simulink model "boost_and_two_level_bridge_rtlab_2_sc_console"  (Simulink 8.4)
settings: Solver=ode3  SolverMode=SingleTasking  StartTime=0.0  StopTime=inf  FixedStep=2e-05  RelTol=1e-3
PostLoadFcn:
  | Ts = 20e-6;
InitFcn:
  | Ts = 20e-6;
libraries: opal_lib x6, simulink x2, efs_cpuhilios_crtl_lib x1
settings Model: ARTEMISmethode_block_infos=$$__separator__$$boost_and_two_level_bridge_rtlab/ARTEMIS Guide$$__separator__$$  Creator=PYRobert  LastModifiedBy=jiang  BufferReuse=off
settings DataIOCC: SaveOutput=off  SignalLogging=off  SaveTime=off  SignalLoggingName=sigsOut
settings OptimizationCC: BlockReduction=off  OptimizeBlockIOStorage=off  BufferReuse=off  GlobalBufferReuse=off  ExpressionFolding=off  LocalBlockOutputs=off  InitFltsAndDblsToZero=on
settings DebuggingCC: SaveWithParameterizedLinksMsg=none  SignalResolutionControl=TryResolveAllWithWarning  SolverPrmCheckMsg=none  MultiTaskDSMMsg=warning  MultiTaskCondExecSysMsg=none
settings HardwareCC: TargetEndianess=LittleEndian  TargetHWDeviceType=MATLAB Host  ProdEqTarget=off
settings RTWCC: GenCodeOnly=on  IncludeERTFirstTime=on
settings GRTTargetCC: TargetFcnLib=ansi_tfl_tmw.mat
settings ConfigurationSet: Description=SimMechanics 2G

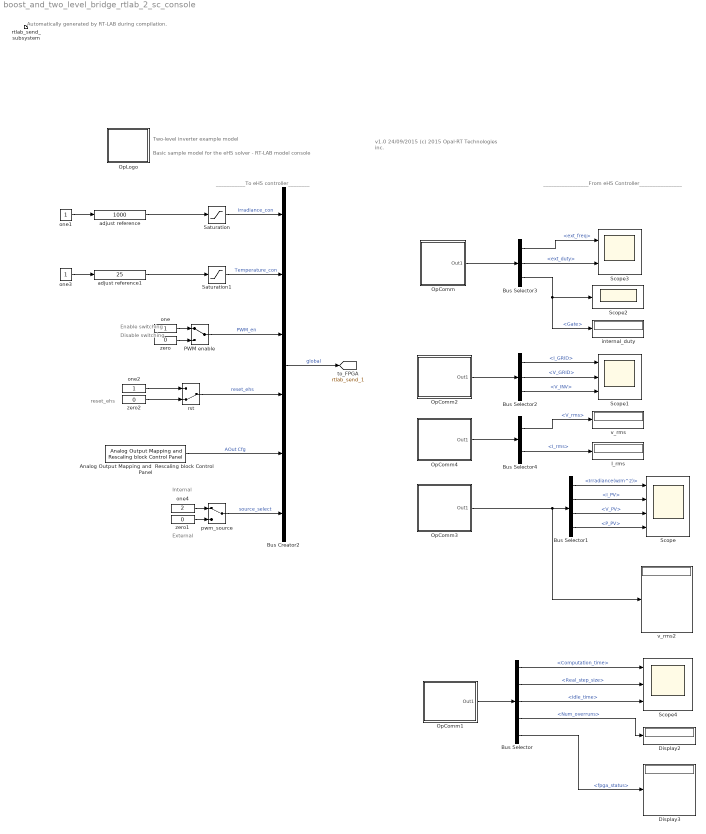
== system boost_and_two_level_bridge_rtlab_2_sc_console ==
  note: reset_ehs
  note: Basic sample model for the eHS solver - RT-LAB model console
  note: Two-level inverter example model
  note: v1.0 24/09/2015
      | (c) 2015 Opal-RT Technologies inc.
  note: Disable switching
  note: Enable switching
  note: _________________From eHS Controller________________
  note: ___________To eHS controller________
  note: Internal
  note: External
  note: Automatically generated by RT-LAB during compilation.
  Analog Output Mapping and  Rescaling block Control Panel : efs_cpuhilios_crtl_lib/Analog Output Mapping and  Rescaling block Control Panel  NbChannels=32  SigNames={'eHS.Y01' 'eHS.Y02' 'eHS.Y03' 'eHS.Y04' 'eHS.Y05' 'eHS.Y06' 'eHS.Y07' 'eHS.Y08' 'eHS.Y09' 'eHS.Y10' 'eHS.Y11' 'eHS.Y12' 'eHS.Y13' 'eHS.Y14' 'eHS.Y15' 'eHS.Y16' 'eHS.Y17' 'eHS.Y18' 'eHS.Y19' 'eHS.Y20' 'eHS.Y21' 'eHS.Y22' 'eHS.Y23' 'eHS.Y24' 'eHS.Y25' 'eHS.Y26' 'eHS.Y27' 'eHS.Y28' 'eHS.Y29' 'eHS.Y30' 'eHS.Y31' 'eHS.Y32'}  NbUsrAOut=16  signalch0=User2  signalch1=User1  signalch2=User5  signalch3=User6  signalch4=User6  signalch5=eHS.Y10  signalch6=eHS.Y02  signalch7=eHS.Y04  signalch8=eHS.Y13  signalch9=eHS.Y14  signalch10=eHS.Y01  signalch11=eHS.Y03  signalch12=User1  signalch13=User2  signalch14=User3  signalch15=User4  signalch16=User1  signalch17=User2  signalch18=User3  signalch19=User4  signalch20=User5  signalch21=User6  signalch22=User7  signalch23=User7  signalch24=User9  signalch25=User10  signalch26=User11  signalch27=User12  signalch28=User13  signalch29=User14  signalch30=User15  signalch31=User16  gain0=0.0066  gain1=0.33  gain2=0.066  gain3=0.0041250  gain4=0.0048529  gain5=1  gain6=0.005  gain7=0.005  gain8=0.1  gain9=0.1  gain10=0.1  gain11=0.1  gain12=.005  gain13=.1  gain14=.1  gain15=.1  gain16=1  gain17=1  gain18=1  gain19=1  gain20=1  gain21=1  gain22=1  gain23=1  gain24=1  gain25=1  gain26=1  gain27=1  gain28=1  gain29=1  gain30=1  gain31=1  offset0=0  offset1=0  offset2=1.65  offset3=1.6500  offset4=1.6500  offset5=0  offset6=0  offset7=0  offset8=0  offset9=0  offset10=0  offset11=0  offset12=0  offset13=0  offset14=0  offset15=0  offset16=0  offset17=0  offset18=0  offset19=0  offset20=0  offset21=0  offset22=0  offset23=0  offset24=0  offset25=0  offset26=0  offset27=0  offset28=0  offset29=0  offset30=0  offset31=0  max0=3.3  max1=3.3  max2=3.3  max3=3.3  max4=3.3  max5=5  max6=5  max7=5  max8=5  max9=5  max10=5  max11=5  max12=16  max13=16  max14=16  max15=16  max16=16  max17=16  max18=16  max19=16  max20=16  max21=16  max22=16  max23=16  max24=16  max25=16  max26=16  max27=16  max28=16  max29=16  max30=16  max31=16  min0=0  min1=0  min2=0  min3=0  min4=0  min5=-5  min6=-5  min7=-5  min8=-5  min9=-5  min10=-5  min11=-5  min12=-16  min13=-16  min14=-16  min15=-16  min16=-16  min17=-16  min18=-16  min19=-16  min20=-16  min21=-16  min22=-16  min23=-16  min24=-16  min25=-16  min26=-16  min27=-16  min28=-16  min29=-16  min30=-16  min31=-16  map=[ 49 48 52 53 53 9 1 3 12 13 0 2 48 49 50 51 48 49 50 51 52 53 54 54 56 57 58 59 60 61 62 63 ]
      link override Display2: Decimation=12500
  Bus Creator2 : BusCreator  Inputs=6
  Bus Selector : BusSelector  OutputSignals=Computation_time,Real_step_size,Idle_time,Num_overruns,fpga_status
  Bus Selector1 : BusSelector  OutputSignals=Irradiance(w/m^2),I_PV,V_PV,P_PV
  Bus Selector2 : BusSelector  OutputSignals=I_GRID,V_GRID,V_INV
  Bus Selector3 : BusSelector  OutputSignals=digital_in.ext_freq,digital_in.ext_duty,Gate
  Bus Selector4 : BusSelector  OutputSignals=V_rms,I_rms
  Display2 : Display
      settings: Decimation=12500
  Display3 : Display
      settings: Decimation=12500
  I_rms : Display
      settings: Decimation=12500
  OpComm : Subsystem
      mask init:
      | opmaskdisplay('maskdisplay_block',gcb,'disp(''OpComm'')');
      mask Display:
      | patch([0 0.5 0.7 0],[1 1 0 0],[0.7 0.75 0.9]);
      | patch([1 0.53 0.73 1],[1 1 0 0],[1 0.8 0.7]);
      | plot([0 0 1 1 0],[0 1 1 0 0]);
      | disp('OpComm')
  OpComm1 : Subsystem
      mask init:
      | opmaskdisplay('maskdisplay_block',gcb,'disp(''OpComm'')');
      mask Display:
      | patch([0 0.5 0.7 0],[1 1 0 0],[0.7 0.75 0.9]);
      | patch([1 0.53 0.73 1],[1 1 0 0],[1 0.8 0.7]);
      | plot([0 0 1 1 0],[0 1 1 0 0]);
      | disp('OpComm')
  OpComm2 : Subsystem
      mask init:
      | opmaskdisplay('maskdisplay_block',gcb,'disp(''OpComm'')');
      mask Display:
      | patch([0 0.5 0.7 0],[1 1 0 0],[0.7 0.75 0.9]);
      | patch([1 0.53 0.73 1],[1 1 0 0],[1 0.8 0.7]);
      | plot([0 0 1 1 0],[0 1 1 0 0]);
      | disp('OpComm')
  OpComm3 : Subsystem
      mask init:
      | opmaskdisplay('maskdisplay_block',gcb,'disp(''OpComm'')');
      mask Display:
      | patch([0 0.5 0.7 0],[1 1 0 0],[0.7 0.75 0.9]);
      | patch([1 0.53 0.73 1],[1 1 0 0],[1 0.8 0.7]);
      | plot([0 0 1 1 0],[0 1 1 0 0]);
      | disp('OpComm')
  OpComm4 : Subsystem
      mask init:
      | opmaskdisplay('maskdisplay_block',gcb,'disp(''OpComm'')');
      mask Display:
      | patch([0 0.5 0.7 0],[1 1 0 0],[0.7 0.75 0.9]);
      | patch([1 0.53 0.73 1],[1 1 0 0],[1 0.8 0.7]);
      | plot([0 0 1 1 0],[0 1 1 0 0]);
      | disp('OpComm')
  OpLogo : Subsystem
      mask Display:
      | opLogo = imread('efsOpLogo.tif','tif');
      | image(opLogo(:,:,1:3));
  PWM enable : ManualSwitch
  Saturation : Saturate  UpperLimit=1000  LowerLimit=0
  Saturation1 : Saturate  UpperLimit=60  LowerLimit=-10
  Scope : Scope  NumInputPorts=4
      settings: YMin=-5~-5~-5~-5  YMax=5~5~5~5  Decimation=100  SampleInput=on  SampleTime=2e-3
  Scope1 : Scope  NumInputPorts=3
      settings: YMin=-500~-400~-800  YMax=500~400~800  SaveName=ScopeData2  SampleInput=on  SampleTime=1e-3
  Scope2 : Scope
      settings: YMin=0  YMax=1  SaveName=ScopeData3  MaxDataPoints=10000  SampleInput=on  SampleTime=2e-4
  Scope3 : Scope  NumInputPorts=2
      settings: YMin=-5~-5  YMax=5~5  SaveName=ScopeData4  MaxDataPoints=100000  SampleInput=on  SampleTime=1e-3
  Scope4 : Scope  NumInputPorts=3
      settings: YMin=-5~-5~-5  YMax=5~5~5  SaveName=ScopeData5  SampleInput=on  SampleTime=5e-2
  adjust reference : simulink/Math Operations/Slider Gain  low=0  gain=1000  high=1000
  adjust reference1 : simulink/Math Operations/Slider Gain  low=0  gain=25  high=60
  internal_duty : Display
      settings: Decimation=12500
  one{,1..3} (4 alike) : Constant
  one4 : Constant  Value=2
  pwm_source : ManualSwitch
  rst : ManualSwitch  CurrentSetting=0
  rtlab_send_subsystem : Subsystem  Priority=-100
      mask Display: text(0,0,'');
  v_rms : Display
      settings: Decimation=12500
  v_rms2 : Display
      settings: Decimation=12500
  zero : Constant  Value=0
  zero1 : Constant  Value=0
  zero2 : Constant  Value=0
  tag scope: rtlab_send_1=global
  wires:
  Bus Selector4/2 -> I_rms/1  "<I_rms>"
  Bus Selector4/1 -> v_rms/1  "<V_rms>"
  OpComm4/1(Out1) -> Bus Selector4/1
  Bus Selector/5 -> Display3/1  "<fpga_status>"
  Bus Selector3/3 -> Scope2/1, internal_duty/1  "<Gate>"
  Bus Selector3/2 -> Scope3/2  "<ext_duty>"
  Bus Selector3/1 -> Scope3/1  "<ext_freq>"
  OpComm/1(Out1) -> Bus Selector3/1
  Bus Selector2/3 -> Scope1/3  "<V_INV>"
  Bus Selector2/1 -> Scope1/1  "<I_GRID>"
  Bus Selector2/2 -> Scope1/2  "<V_GRID>"
  OpComm2/1(Out1) -> Bus Selector2/1
  Bus Selector1/3 -> Scope/3  "<V_PV>"
  Bus Selector1/4 -> Scope/4  "<P_PV>"
  Bus Selector1/2 -> Scope/2  "<I_PV>"
  Bus Selector1/1 -> Scope/1  "<Irradiance(w/m^2)>"
  OpComm3/1(Out1) -> v_rms2/1, Bus Selector1/1
  OpComm1/1(Out1) -> Bus Selector/1
  pwm_source/1 -> Bus Creator2/6  "source_select"
  one4/1 -> pwm_source/1
  zero1/1 -> pwm_source/2
  Analog Output Mapping and  Rescaling block Control Panel/1 -> Bus Creator2/5  "AOut Cfg"
  Bus Selector/1 -> Scope4/1  "<Computation_time>"
  Bus Selector/4 -> Display2/1  "<Num_overruns>"
  Bus Selector/2 -> Scope4/2  "<Real_step_size>"
  Bus Selector/3 -> Scope4/3  "<Idle_time>"
  Saturation1/1 -> Bus Creator2/2  "Temperature_con"
  Saturation/1 -> Bus Creator2/1  "Irradiance_con"
  adjust reference1/1 -> Saturation1/1
  adjust reference/1 -> Saturation/1
  one3/1 -> adjust reference1/1
  one1/1 -> adjust reference/1
  one2/1 -> rst/1
  zero2/1 -> rst/2
  rst/1 -> Bus Creator2/4  "reset_ehs"
  one/1 -> PWM enable/1
  zero/1 -> PWM enable/2
  PWM enable/1 -> Bus Creator2/3  "PWM_en"
  Bus Creator2/1 -> [rtlab_send_1]  "global"

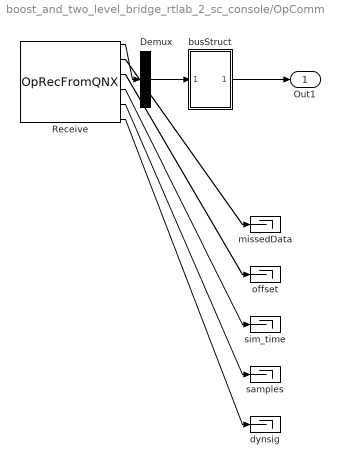
== system boost_and_two_level_bridge_rtlab_2_sc_console/OpComm ==
  Demux : Demux  Outputs=[4]
  Receive : opal_lib/Communication/OpRecFromQNX  Node_num=1  Acqu_Group=1  Data_Width=4  Synchronization=on  Interpolation=on  Threshold=1.0  modelname=boost_and_two_level_bridge_rtlab.mdl  sampletime=2e-05
  busStruct : Subsystem
  dynsig : Terminator
  missedData : Terminator
  offset : Terminator
  samples : Terminator
  sim_time : Terminator
  Out1 : Outport
  wires:
  Demux/1 -> busStruct/1(In1)
  busStruct/1(Out1) -> Out1/1
  Receive/1 -> Demux/1
  Receive/6 -> dynsig/1
  Receive/5 -> samples/1
  Receive/4 -> sim_time/1
  Receive/3 -> offset/1
  Receive/2 -> missedData/1

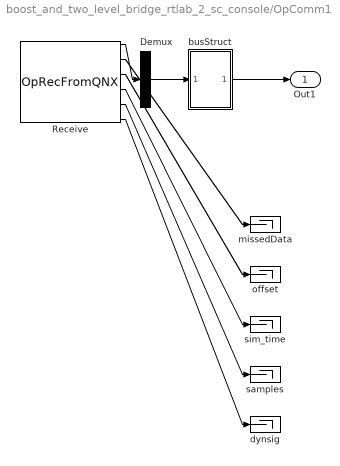
== system boost_and_two_level_bridge_rtlab_2_sc_console/OpComm1 ==
  Demux : Demux  Outputs=[8]
  Receive : opal_lib/Communication/OpRecFromQNX  Node_num=1  Acqu_Group=2  Data_Width=8  Synchronization=on  Interpolation=on  Threshold=1.0  modelname=boost_and_two_level_bridge_rtlab.mdl  sampletime=2e-05
  busStruct : Subsystem
  dynsig : Terminator
  missedData : Terminator
  offset : Terminator
  samples : Terminator
  sim_time : Terminator
  Out1 : Outport
  wires:
  Demux/1 -> busStruct/1(In1)
  busStruct/1(Out1) -> Out1/1
  Receive/1 -> Demux/1
  Receive/6 -> dynsig/1
  Receive/5 -> samples/1
  Receive/4 -> sim_time/1
  Receive/3 -> offset/1
  Receive/2 -> missedData/1

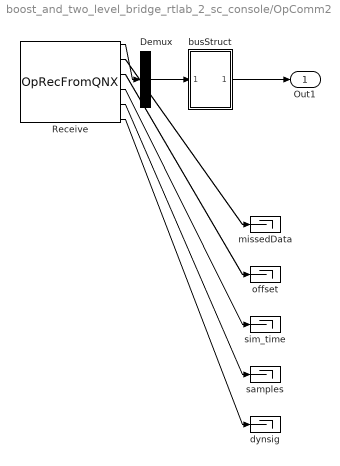
== system boost_and_two_level_bridge_rtlab_2_sc_console/OpComm2 ==
  Demux : Demux  Outputs=[3]
  Receive : opal_lib/Communication/OpRecFromQNX  Node_num=1  Acqu_Group=4  Data_Width=3  Synchronization=on  Interpolation=on  Threshold=1.0  modelname=boost_and_two_level_bridge_rtlab.mdl  sampletime=2e-05
  busStruct : Subsystem
  dynsig : Terminator
  missedData : Terminator
  offset : Terminator
  samples : Terminator
  sim_time : Terminator
  Out1 : Outport
  wires:
  Demux/1 -> busStruct/1(In1)
  busStruct/1(Out1) -> Out1/1
  Receive/1 -> Demux/1
  Receive/6 -> dynsig/1
  Receive/5 -> samples/1
  Receive/4 -> sim_time/1
  Receive/3 -> offset/1
  Receive/2 -> missedData/1

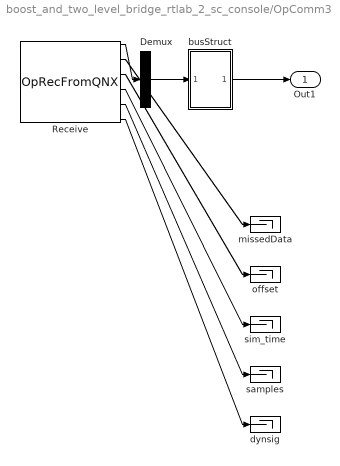
== system boost_and_two_level_bridge_rtlab_2_sc_console/OpComm3 ==
  Demux : Demux  Outputs=[6]
  Receive : opal_lib/Communication/OpRecFromQNX  Node_num=1  Acqu_Group=3  Data_Width=6  Synchronization=on  Interpolation=on  Threshold=1.0  modelname=boost_and_two_level_bridge_rtlab.mdl  sampletime=2e-05
  busStruct : Subsystem
  dynsig : Terminator
  missedData : Terminator
  offset : Terminator
  samples : Terminator
  sim_time : Terminator
  Out1 : Outport
  wires:
  Demux/1 -> busStruct/1(In1)
  busStruct/1(Out1) -> Out1/1
  Receive/1 -> Demux/1
  Receive/6 -> dynsig/1
  Receive/5 -> samples/1
  Receive/4 -> sim_time/1
  Receive/3 -> offset/1
  Receive/2 -> missedData/1

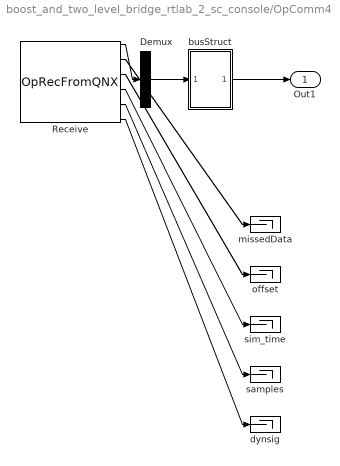
== system boost_and_two_level_bridge_rtlab_2_sc_console/OpComm4 ==
  Demux : Demux  Outputs=[2]
  Receive : opal_lib/Communication/OpRecFromQNX  Node_num=1  Acqu_Group=5  Data_Width=2  Synchronization=on  Interpolation=on  Threshold=1.0  modelname=boost_and_two_level_bridge_rtlab.mdl  sampletime=2e-05
  busStruct : Subsystem
  dynsig : Terminator
  missedData : Terminator
  offset : Terminator
  samples : Terminator
  sim_time : Terminator
  Out1 : Outport
  wires:
  Demux/1 -> busStruct/1(In1)
  busStruct/1(Out1) -> Out1/1
  Receive/1 -> Demux/1
  Receive/6 -> dynsig/1
  Receive/5 -> samples/1
  Receive/4 -> sim_time/1
  Receive/3 -> offset/1
  Receive/2 -> missedData/1

== system boost_and_two_level_bridge_rtlab_2_sc_console/OpLogo ==

== system boost_and_two_level_bridge_rtlab_2_sc_console/rtlab_send_subsystem ==
  Subsystem6 : Subsystem
  wires:
  [rtlab_send_1] -> Subsystem6/1(In1)

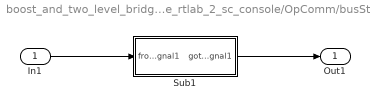
== system boost_and_two_level_bridge_rtlab_2_sc_console/OpComm/busStruct ==
  In1 : Inport
  Sub1 : Subsystem
  Out1 : Outport
  wires:
  Sub1/1(goto_signal1) -> Out1/1
  In1/1 -> Sub1/1(from_signal1)

== system boost_and_two_level_bridge_rtlab_2_sc_console/OpComm1/busStruct ==
  In1 : Inport
  Sub1 : Subsystem
  Out1 : Outport
  wires:
  Sub1/1(goto_signal1) -> Out1/1
  In1/1 -> Sub1/1(from_signal1)

== system boost_and_two_level_bridge_rtlab_2_sc_console/OpComm2/busStruct ==
  In1 : Inport
  Sub1 : Subsystem
  Out1 : Outport
  wires:
  Sub1/1(goto_signal1) -> Out1/1
  In1/1 -> Sub1/1(from_signal1)

== system boost_and_two_level_bridge_rtlab_2_sc_console/OpComm3/busStruct ==
  In1 : Inport
  Sub1 : Subsystem
  Out1 : Outport
  wires:
  Sub1/1(goto_signal1) -> Out1/1
  In1/1 -> Sub1/1(from_signal1)

== system boost_and_two_level_bridge_rtlab_2_sc_console/OpComm4/busStruct ==
  In1 : Inport
  Sub1 : Subsystem
  Out1 : Outport
  wires:
  Sub1/1(goto_signal1) -> Out1/1
  In1/1 -> Sub1/1(from_signal1)

== system boost_and_two_level_bridge_rtlab_2_sc_console/rtlab_send_subsystem/Subsystem6 ==
  In1 : Inport  PortDimensions=165
  Mux : Mux  Inputs=1
  Send6 : opal_lib/Communication/OpSendPar ToQNX  Node_num=1  modelname=boost_and_two_level_bridge_rtlab
  wires:
  Mux/1 -> Send6/1
  In1/1 -> Mux/1

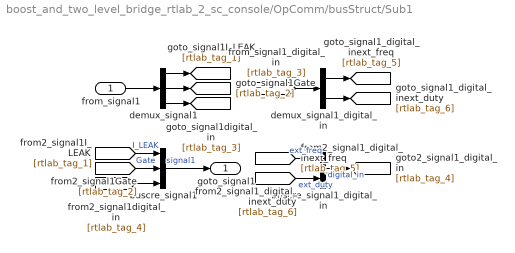
== system boost_and_two_level_bridge_rtlab_2_sc_console/OpComm/busStruct/Sub1 ==
  from_signal1 : Inport
  buscre_signal1 : BusCreator  Inputs=3
  buscre_signal1_digital_in : BusCreator  Inputs=2
  demux_signal1 : Demux  Outputs="[1  1  2]"
  demux_signal1_digital_in : Demux  Outputs="[1  1]"
  goto_signal1 : Outport
  wires:
  buscre_signal1_digital_in/1 -> [rtlab_tag_4]  "digital_in"
  [rtlab_tag_6] -> buscre_signal1_digital_in/2  "ext_duty"
  [rtlab_tag_5] -> buscre_signal1_digital_in/1  "ext_freq"
  demux_signal1_digital_in/2 -> [rtlab_tag_6]
  demux_signal1_digital_in/1 -> [rtlab_tag_5]
  [rtlab_tag_3] -> demux_signal1_digital_in/1
  buscre_signal1/1 -> goto_signal1/1  "signal1"
  [rtlab_tag_4] -> buscre_signal1/3
  [rtlab_tag_2] -> buscre_signal1/2  "Gate"
  [rtlab_tag_1] -> buscre_signal1/1  "I_LEAK"
  demux_signal1/3 -> [rtlab_tag_3]
  demux_signal1/2 -> [rtlab_tag_2]
  demux_signal1/1 -> [rtlab_tag_1]
  from_signal1/1 -> demux_signal1/1

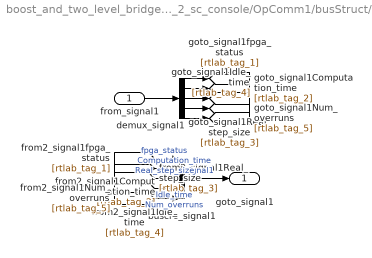
== system boost_and_two_level_bridge_rtlab_2_sc_console/OpComm1/busStruct/Sub1 ==
  from_signal1 : Inport
  buscre_signal1 : BusCreator  Inputs=5
  demux_signal1 : Demux  Outputs="[4  1  1  1  1]"
  goto_signal1 : Outport
  wires:
  buscre_signal1/1 -> goto_signal1/1  "signal1"
  [rtlab_tag_5] -> buscre_signal1/5  "Num_overruns"
  [rtlab_tag_4] -> buscre_signal1/4  "Idle_time"
  [rtlab_tag_3] -> buscre_signal1/3  "Real_step_size"
  [rtlab_tag_2] -> buscre_signal1/2  "Computation_time"
  [rtlab_tag_1] -> buscre_signal1/1  "fpga_status"
  demux_signal1/5 -> [rtlab_tag_5]
  demux_signal1/4 -> [rtlab_tag_4]
  demux_signal1/3 -> [rtlab_tag_3]
  demux_signal1/2 -> [rtlab_tag_2]
  demux_signal1/1 -> [rtlab_tag_1]
  from_signal1/1 -> demux_signal1/1

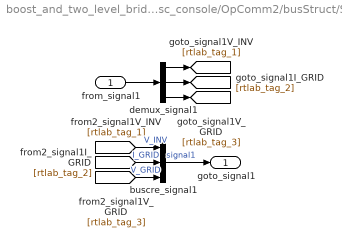
== system boost_and_two_level_bridge_rtlab_2_sc_console/OpComm2/busStruct/Sub1 ==
  from_signal1 : Inport
  buscre_signal1 : BusCreator  Inputs=3
  demux_signal1 : Demux  Outputs="[1  1  1]"
  goto_signal1 : Outport
  wires:
  buscre_signal1/1 -> goto_signal1/1  "signal1"
  [rtlab_tag_3] -> buscre_signal1/3  "V_GRID"
  [rtlab_tag_2] -> buscre_signal1/2  "I_GRID"
  [rtlab_tag_1] -> buscre_signal1/1  "V_INV"
  demux_signal1/3 -> [rtlab_tag_3]
  demux_signal1/2 -> [rtlab_tag_2]
  demux_signal1/1 -> [rtlab_tag_1]
  from_signal1/1 -> demux_signal1/1

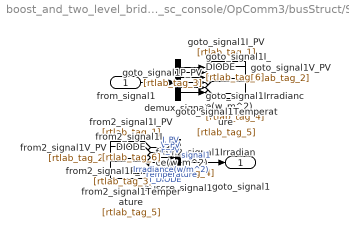
== system boost_and_two_level_bridge_rtlab_2_sc_console/OpComm3/busStruct/Sub1 ==
  from_signal1 : Inport
  buscre_signal1 : BusCreator  Inputs=6
  demux_signal1 : Demux  Outputs="[1  1  1  1  1  1]"
  goto_signal1 : Outport
  wires:
  buscre_signal1/1 -> goto_signal1/1  "signal1"
  [rtlab_tag_6] -> buscre_signal1/6  "I_DIODE"
  [rtlab_tag_5] -> buscre_signal1/5  "Temperature"
  [rtlab_tag_4] -> buscre_signal1/4  "Irradiance(w/m^2)"
  [rtlab_tag_3] -> buscre_signal1/3  "P_PV"
  [rtlab_tag_2] -> buscre_signal1/2  "V_PV"
  [rtlab_tag_1] -> buscre_signal1/1  "I_PV"
  demux_signal1/6 -> [rtlab_tag_6]
  demux_signal1/5 -> [rtlab_tag_5]
  demux_signal1/4 -> [rtlab_tag_4]
  demux_signal1/3 -> [rtlab_tag_3]
  demux_signal1/2 -> [rtlab_tag_2]
  demux_signal1/1 -> [rtlab_tag_1]
  from_signal1/1 -> demux_signal1/1

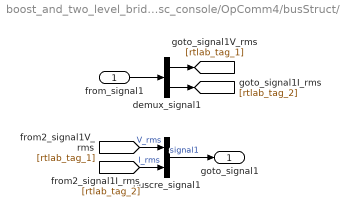
== system boost_and_two_level_bridge_rtlab_2_sc_console/OpComm4/busStruct/Sub1 ==
  from_signal1 : Inport
  buscre_signal1 : BusCreator  Inputs=2
  demux_signal1 : Demux  Outputs="[1  1]"
  goto_signal1 : Outport
  wires:
  buscre_signal1/1 -> goto_signal1/1  "signal1"
  [rtlab_tag_2] -> buscre_signal1/2  "I_rms"
  [rtlab_tag_1] -> buscre_signal1/1  "V_rms"
  demux_signal1/2 -> [rtlab_tag_2]
  demux_signal1/1 -> [rtlab_tag_1]
  from_signal1/1 -> demux_signal1/1
